simulink model "Vehicle_definitivo_validazione_2"  (R2025b)
settings: Solver=ode4  StartTime=0.0  StopTime=30  FixedStep=0.001  RelTol=1e-3
undefined symbols (not defined in the file): car, new_lotus_bump, new_lotus_roll, new_lotus_steer, posRef, rad, s, Tau_1, Tau_2, Tau_3, Tau_4, yawRef
libraries: aerolibconvert2 x28, simulink_extras x16, simulink x12, slpidlib x2, mpclib x1
(part 10 of 13)

== system Vehicle_definitivo_validazione_2/Torque Vectoring/Vehicle/Chassis/kinematics/FR ==
  note: mettere 2d su cmaber e toe
  Wheel_Travel : Inport
  Steer_Angle : Inport  Port=2
  Add : Sum
  Add1 : Sum  Inputs=+++
  Anti_dive : Lookup_n-D  NumberOfTableDimensions=1  BreakpointsForDimension1=[-20;-19;-18;-17;-16;-15;-14;-13;-12;-11;-10;-9;-8;-7;-6;-5;-4;-3;-2;-1;0;1;2;3;4;5;6;7;8;9;10;11;12;13;14;15;16;17;18;19;20;21;22;23;24;25;26;27;28;29;30;31;32;33;34;35;36;37;38;39;40;41;42;43;44;45;46;47;48;49;50;51;52;53;54;55;56;57;58;59;60;61;62;63;64;65;66;67;68;69;70;71;72;73;74;75]  Table=[53.85;54.03;54.22;54.4;54.59;54.77;54.96;55.15;55.34;55.53;55.72;55.92;56.11;56.31;56.5;56.7;56.9;57.1;57.3;57.5;57.71;57.91;58.12;58.32;58.53;58.74;58.95;59.16;59.38;59.59;59.81;60.03;60.24;60.46;60.69;60.91;61.13;61.36;61.59;61.81;62.04;62.28;62.51;62.74;62.98;63.22;63.46;63.7;63.94;64.18000000000001;64.43000000000001;64.68000000000001;64.92;65.17;65.43000000000001;65.68000000000001;65.94;66.19;66.45;66.72;66.98;67.23999999999999;67.51000000000001;67.78;68.05;68.31999999999999;68.59999999999999;68.87;69.15000000000001;69.43000000000001;69.72;70;70.29000000000001;70.58;70.87;71.16;71.45999999999999;71.75;72.05;72.36;72.66;72.97;73.28;73.59;73.91;74.22;74.54000000000001;74.86;75.19;75.52;75.84999999999999;76.18000000000001;76.51000000000001;76.84999999999999;77.19;77.54000000000001]/100  InternalRulePriority=Speed  RndMeth=Simplest
  Constant : Constant  Value=car.camber0_front
  Constant1 : Constant  Value=car.toe0_front
  Gain : Gain  Gain=0.222222
  IR : Lookup_n-D  NumberOfTableDimensions=1  BreakpointsForDimension1=[-20;-19;-18;-17;-16;-15;-14;-13;-12;-11;-10;-9;-8;-7;-6;-5;-4;-3;-2;-1;0;1;2;3;4;5;6;7;8;9;10;11;12;13;14;15;16;17;18;19;20;21;22;23;24;25;26;27;28;29;30;31;32;33;34;35;36;37;38;39;40;41;42;43;44;45;46;47;48;49;50;51;52;53;54;55;56;57;58;59;60;61;62;63;64;65;66;67;68;69;70;71;72;73;74;75]  Table=[0.556793;0.557414;0.558036;0.558659;0.559284;0.55991;0.5602240000000001;0.560538;0.561167;0.561167;0.561482;0.561798;0.562114;0.562114;0.562114;0.562114;0.562114;0.562114;0.562114;0.562114;0.561798;0.561798;0.561482;0.561482;0.561167;0.560852;0.560538;0.5602240000000001;0.55991;0.559284;0.558971;0.558347;0.558036;0.557414;0.557103;0.5564829999999999;0.555864;0.555247;0.554631;0.554017;0.553403;0.552792;0.552181;0.551572;0.550661;0.550055;0.549451;0.548546;0.547945;0.547046;0.546448;0.545554;0.544662;0.543774;0.543183;0.542299;0.541419;0.540541;0.539665;0.538793;0.537924;0.537057;0.536193;0.535332;0.534474;0.533618;0.532765;0.531915;0.531067;0.529942;0.529101;0.528262;0.527426;0.526593;0.525486;0.524659;0.523834;0.522739;0.521921;0.521105;0.5202909999999999;0.519211;0.5184029999999999;0.517598;0.516529;0.51573;0.514933;0.514139;0.513084;0.5122949999999999;0.511509;0.510725;0.509944;0.509165;0.508388;0.507614]  InternalRulePriority=Speed  RndMeth=Simplest
  camber : Lookup_n-D  NumberOfTableDimensions=1  BreakpointsForDimension1=[-20;-19;-18;-17;-16;-15;-14;-13;-12;-11;-10;-9;-8;-7;-6;-5;-4;-3;-2;-1;0;1;2;3;4;5;6;7;8;9;10;11;12;13;14;15;16;17;18;19;20;21;22;23;24;25;26;27;28;29;30;31;32;33;34;35;36;37;38;39;40;41;42;43;44;45;46;47;48;49;50;51;52;53;54;55;56;57;58;59;60;61;62;63;64;65;66;67;68;69;70;71;72;73;74;75]  Table=[0.17;0.13;0.08;0.04;-0.01;-0.05;-0.1;-0.15;-0.19;-0.24;-0.29;-0.33;-0.38;-0.42;-0.47;-0.52;-0.5600000000000001;-0.61;-0.66;-0.7;-0.75;-0.8;-0.84;-0.89;-0.9399999999999999;-0.98;-1.03;-1.08;-1.13;-1.17;-1.22;-1.27;-1.31;-1.36;-1.41;-1.46;-1.5;-1.55;-1.6;-1.65;-1.7;-1.74;-1.79;-1.84;-1.89;-1.94;-1.99;-2.03;-2.08;-2.13;-2.18;-2.23;-2.28;-2.33;-2.38;-2.42;-2.47;-2.52;-2.57;-2.62;-2.67;-2.72;-2.77;-2.82;-2.87;-2.92;-2.97;-3.02;-3.07;-3.12;-3.17;-3.23;-3.28;-3.33;-3.38;-3.43;-3.48;-3.53;-3.58;-3.64;-3.69;-3.74;-3.79;-3.84;-3.9;-3.95;-4;-4.05;-4.11;-4.16;-4.21;-4.27;-4.32;-4.37;-4.43;-4.48]+0.75  InternalRulePriority=Speed  RndMeth=Simplest
  steer vs toe : Lookup_n-D  NumberOfTableDimensions=1  BreakpointsForDimension1=new_lotus_steer.rack_travel  Table=new_lotus_steer.toe_angle_LHS  InternalRulePriority=Speed  RndMeth=Simplest
  toe : Lookup_n-D  NumberOfTableDimensions=1  BreakpointsForDimension1=[-20;-19;-18;-17;-16;-15;-14;-13;-12;-11;-10;-9;-8;-7;-6;-5;-4;-3;-2;-1;0;1;2;3;4;5;6;7;8;9;10;11;12;13;14;15;16;17;18;19;20;21;22;23;24;25;26;27;28;29;30;31;32;33;34;35;36;37;38;39;40;41;42;43;44;45;46;47;48;49;50;51;52;53;54;55;56;57;58;59;60;61;62;63;64;65;66;67;68;69;70;71;72;73;74;75]  Table=new_lotus_bump.front_LHS.toe  InternalRulePriority=Speed  RndMeth=Simplest
  wheelbase_change : Lookup_n-D  NumberOfTableDimensions=1  BreakpointsForDimension1=[-20;-19;-18;-17;-16;-15;-14;-13;-12;-11;-10;-9;-8;-7;-6;-5;-4;-3;-2;-1;0;1;2;3;4;5;6;7;8;9;10;11;12;13;14;15;16;17;18;19;20;21;22;23;24;25;26;27;28;29;30;31;32;33;34;35;36;37;38;39;40;41;42;43;44;45;46;47;48;49;50;51;52;53;54;55;56;57;58;59;60;61;62;63;64;65;66;67;68;69;70;71;72;73;74;75]  Table=[0.68000000000000005;0.65000000000000002;0.60999999999999999;0.56999999999999995;0.54000000000000004;0.5;0.46999999999999997;0.42999999999999999;0.40000000000000002;0.35999999999999999;0.33000000000000002;0.28999999999999998;0.26000000000000001;0.23000000000000001;0.19;0.16;0.13;0.089999999999999997;0.059999999999999998;0.029999999999999999;0;-0.029999999999999999;-0.059999999999999998;-0.089999999999999997;-0.12;-0.14999999999999999;-0.17999999999999999;-0.20999999999999999;-0.23999999999999999;-0.27000000000000002;-0.29999999999999999;-0.32000000000000001;-0.34999999999999998;-0.38;-0.40000000000000002;-0.42999999999999999;-0.46000000000000002;-0.47999999999999998;-0.51000000000000001;-0.53000000000000003;-0.56000000000000005;-0.57999999999999996;-0.60999999999999999;-0.63;-0.65000000000000002;-0.68000000000000005;-0.69999999999999996;-0.71999999999999997;-0.73999999999999999;-0.76000000000000001;-0.79000000000000004;-0.81000000000000005;-0.82999999999999996;-0.84999999999999998;-0.87;-0.89000000000000001;-0.91000000000000003;-0.92000000000000004;-0.93999999999999995;-0.95999999999999996;-0.97999999999999998;-0.98999999999999999;-1.01;-1.03;-1.04;-1.0600000000000001;-1.0700000000000001;-1.0900000000000001;-1.1000000000000001;-1.1200000000000001;-1.1299999999999999;-1.1399999999999999;-1.1499999999999999;-1.1699999999999999;-1.1799999999999999;-1.1899999999999999;-1.2;-1.21;-1.22;-1.23;-1.24;-1.25;-1.26;-1.26;-1.27;-1.28;-1.29;-1.29;-1.3;-1.3;-1.3100000000000001;-1.3100000000000001;-1.3100000000000001;-1.3200000000000001;-1.3200000000000001;-1.3200000000000001]/1000  InternalRulePriority=Speed  RndMeth=Simplest
  wb_FR : Outport
  AD_FR : Outport  Port=2
  IR_FR : Outport  Port=3
  Camber_FR : Outport  Port=4
  Toe_FR : Outport  Port=5
  wires:
  Wheel_Travel/1 -> Anti_dive/1, IR/1, toe/1, camber/1, wheelbase_change/1
  wheelbase_change/1 -> wb_FR/1
  Anti_dive/1 -> AD_FR/1
  IR/1 -> IR_FR/1
  camber/1 -> Add/2
  Constant/1 -> Add/1
  Add/1 -> Camber_FR/1
  Add1/1 -> Toe_FR/1
  Constant1/1 -> Add1/1
  toe/1 -> Add1/2
  steer vs toe/1 -> Add1/3  "toe_FR"
  Gain/1 -> steer vs toe/1
  Steer_Angle/1 -> Gain/1

== system Vehicle_definitivo_validazione_2/Torque Vectoring/Vehicle/Chassis/kinematics/RL ==
  Wheel_Travel : Inport
  Add : Sum
  Add2 : Sum
  Anti_squat : Lookup_n-D  NumberOfTableDimensions=1  BreakpointsForDimension1=[-20;-19;-18;-17;-16;-15;-14;-13;-12;-11;-10;-9;-8;-7;-6;-5;-4;-3;-2;-1;0;1;2;3;4;5;6;7;8;9;10;11;12;13;14;15;16;17;18;19;20;21;22;23;24;25;26;27;28;29;30;31;32;33;34;35;36;37;38;39;40;41;42;43;44;45;46;47;48;49;50;51;52;53;54;55;56;57;58;59;60;61;62;63;64;65;66;67;68;69;70;71;72;73;74;75]  Table=[53.82;53.82;53.82;53.82;53.82;53.82;53.82;53.82;53.82;53.82;53.83;53.83;53.83;53.83;53.84;53.84;53.84;53.85;53.85;53.86;53.86;53.87;53.87;53.88;53.88;53.89;53.9;53.9;53.91;53.92;53.92;53.93;53.94;53.95;53.95;53.96;53.97;53.98;53.99;54;54.01;54.01;54.02;54.03;54.04;54.05;54.06;54.07;54.08;54.09;54.1;54.11;54.12;54.13;54.15;54.16;54.17;54.18;54.19;54.2;54.21;54.22;54.23;54.24;54.25;54.27;54.28;54.29;54.3;54.31;54.32;54.33;54.34;54.35;54.36;54.37;54.38;54.39;54.4;54.41;54.42;54.43;54.44;54.45;54.46;54.47;54.48;54.49;54.49;54.5;54.51;54.52;54.52;54.53;54.54;54.54]/100  InternalRulePriority=Speed  RndMeth=Simplest
  Constant : Constant  Value=car.camber0_rear
  Constant2 : Constant  Value=car.toe0_rear
  Gain2 : Gain  Gain=-1
  IR : Lookup_n-D  NumberOfTableDimensions=1  BreakpointsForDimension1=[-20;-19;-18;-17;-16;-15;-14;-13;-12;-11;-10;-9;-8;-7;-6;-5;-4;-3;-2;-1;0;1;2;3;4;5;6;7;8;9;10;11;12;13;14;15;16;17;18;19;20;21;22;23;24;25;26;27;28;29;30;31;32;33;34;35;36;37;38;39;40;41;42;43;44;45;46;47;48;49;50;51;52;53;54;55;56;57;58;59;60;61;62;63;64;65;66;67;68;69;70;71;72;73;74;75]  Table=[0.7616000000000001;0.7616000000000001;0.7616000000000001;0.7616000000000001;0.7616000000000001;0.7616000000000001;0.7616000000000001;0.7622;0.7622;0.7628;0.7628;0.7634;0.7639;0.7645;0.7651;0.7657;0.7663;0.7669;0.7675;0.768;0.7692;0.7698;0.7704;0.7716;0.7722;0.7734;0.774;0.7746;0.7758;0.7764;0.7776;0.7782;0.7794;0.78;0.7813;0.7819;0.7831;0.7837;0.7849;0.7855;0.7868000000000001;0.7874;0.7886;0.7893;0.7905;0.7911;0.7917999999999999;0.793;0.7937;0.7943;0.7949000000000001;0.7962;0.7968;0.7974;0.7981;0.7987;0.7994;0.8;0.8;0.8006;0.8013;0.8013;0.8018999999999999;0.8018999999999999;0.8026;0.8026;0.8026;0.8026;0.8026;0.8026;0.8026;0.8018999999999999;0.8018999999999999;0.8013;0.8006;0.8;0.7994;0.7987;0.7974;0.7968;0.7955;0.7943;0.7924;0.7911;0.7893;0.7874;0.7849;0.7831;0.7806;0.7776;0.7752;0.7722;0.7685999999999999;0.7651;0.7616000000000001;0.7576000000000001]  InternalRulePriority=Speed  RndMeth=Simplest
  camber : Lookup_n-D  NumberOfTableDimensions=1  BreakpointsForDimension1=[-20;-19;-18;-17;-16;-15;-14;-13;-12;-11;-10;-9;-8;-7;-6;-5;-4;-3;-2;-1;0;1;2;3;4;5;6;7;8;9;10;11;12;13;14;15;16;17;18;19;20;21;22;23;24;25;26;27;28;29;30;31;32;33;34;35;36;37;38;39;40;41;42;43;44;45;46;47;48;49;50;51;52;53;54;55;56;57;58;59;60;61;62;63;64;65;66;67;68;69;70;71;72;73;74;75]  Table=[0.79000000000000004;0.75;0.70999999999999996;0.67000000000000004;0.63;0.58999999999999997;0.55000000000000004;0.51000000000000001;0.46999999999999997;0.42999999999999999;0.39000000000000001;0.34999999999999998;0.31;0.27000000000000002;0.23999999999999999;0.20000000000000001;0.16;0.12;0.080000000000000002;0.040000000000000001;0;-0.040000000000000001;-0.080000000000000002;-0.12;-0.16;-0.20000000000000001;-0.23999999999999999;-0.27000000000000002;-0.31;-0.34999999999999998;-0.39000000000000001;-0.42999999999999999;-0.46999999999999997;-0.51000000000000001;-0.55000000000000004;-0.58999999999999997;-0.63;-0.67000000000000004;-0.70999999999999996;-0.75;-0.79000000000000004;-0.82999999999999996;-0.85999999999999999;-0.90000000000000002;-0.93999999999999995;-0.97999999999999998;-1.02;-1.0600000000000001;-1.1000000000000001;-1.1399999999999999;-1.1799999999999999;-1.22;-1.26;-1.3;-1.3400000000000001;-1.3799999999999999;-1.4199999999999999;-1.46;-1.5;-1.54;-1.5800000000000001;-1.6200000000000001;-1.6599999999999999;-1.7;-1.74;-1.78;-1.8200000000000001;-1.8600000000000001;-1.8999999999999999;-1.9399999999999999;-1.98;-2.02;-2.0699999999999998;-2.1099999999999999;-2.1499999999999999;-2.1899999999999999;-2.23;-2.27;-2.3100000000000001;-2.3500000000000001;-2.3900000000000001;-2.4399999999999999;-2.48;-2.52;-2.5600000000000001;-2.6000000000000001;-2.6400000000000001;-2.6899999999999999;-2.73;-2.77;-2.8100000000000001;-2.8500000000000001;-2.8999999999999999;-2.9399999999999999;-2.98;-3.02]  InternalRulePriority=Speed  RndMeth=Simplest
  toe : Lookup_n-D  NumberOfTableDimensions=1  BreakpointsForDimension1=new_lotus_bump.wheeltravel  Table=new_lotus_bump.rear_LHS.toe  InternalRulePriority=Speed  RndMeth=Simplest
  wheelbase_change : Lookup_n-D  NumberOfTableDimensions=1  BreakpointsForDimension1=[-20;-19;-18;-17;-16;-15;-14;-13;-12;-11;-10;-9;-8;-7;-6;-5;-4;-3;-2;-1;0;1;2;3;4;5;6;7;8;9;10;11;12;13;14;15;16;17;18;19;20;21;22;23;24;25;26;27;28;29;30;31;32;33;34;35;36;37;38;39;40;41;42;43;44;45;46;47;48;49;50;51;52;53;54;55;56;57;58;59;60;61;62;63;64;65;66;67;68;69;70;71;72;73;74;75]  Table=[-2.1899999999999999;-2.0800000000000001;-1.97;-1.8600000000000001;-1.74;-1.6299999999999999;-1.52;-1.4099999999999999;-1.3;-1.1899999999999999;-1.0800000000000001;-0.96999999999999997;-0.85999999999999999;-0.75;-0.65000000000000002;-0.54000000000000004;-0.42999999999999999;-0.32000000000000001;-0.20999999999999999;-0.11;0;0.11;0.20999999999999999;0.32000000000000001;0.41999999999999998;0.53000000000000003;0.63;0.73999999999999999;0.83999999999999997;0.94999999999999996;1.05;1.1599999999999999;1.26;1.3600000000000001;1.47;1.5700000000000001;1.6699999999999999;1.77;1.8700000000000001;1.98;2.0800000000000001;2.1800000000000002;2.2799999999999998;2.3799999999999999;2.48;2.5800000000000001;2.6800000000000002;2.7799999999999998;2.8799999999999999;2.9700000000000002;3.0699999999999998;3.1699999999999999;3.27;3.3700000000000001;3.46;3.5600000000000001;3.6600000000000001;3.7599999999999998;3.8500000000000001;3.9500000000000002;4.04;4.1399999999999997;4.2400000000000002;4.3300000000000001;4.4299999999999997;4.5199999999999996;4.6100000000000003;4.71;4.7999999999999998;4.9000000000000004;4.9900000000000002;5.0800000000000001;5.1799999999999997;5.2699999999999996;5.3600000000000003;5.4500000000000002;5.5499999999999998;5.6399999999999997;5.7300000000000004;5.8200000000000003;5.9100000000000001;6;6.0899999999999999;6.1799999999999997;6.2699999999999996;6.3600000000000003;6.4500000000000002;6.54;6.6299999999999999;6.7199999999999998;6.8099999999999996;6.9000000000000004;6.9900000000000002;7.0700000000000003;7.1600000000000001;7.25]/1000  InternalRulePriority=Speed  RndMeth=Simplest
  wb_RL : Outport
  AS_RL : Outport  Port=2
  IR_RL : Outport  Port=3
  Camber_RL : Outport  Port=4
  Toe_RL : Outport  Port=5
  wires:
  Wheel_Travel/1 -> Anti_squat/1, wheelbase_change/1, IR/1, toe/1, camber/1
  wheelbase_change/1 -> wb_RL/1
  Anti_squat/1 -> AS_RL/1
  IR/1 -> IR_RL/1
  Add/1 -> Camber_RL/1
  Constant/1 -> Add/1
  camber/1 -> Add/2
  Constant2/1 -> Add2/1
  Add2/1 -> Toe_RL/1
  toe/1 -> Gain2/1
  Gain2/1 -> Add2/2

== system Vehicle_definitivo_validazione_2/Torque Vectoring/Vehicle/Chassis/kinematics/RR ==
  Wheel_Travel : Inport
  Add : Sum
  Add2 : Sum
  Anti_squat : Lookup_n-D  NumberOfTableDimensions=1  BreakpointsForDimension1=[-20;-19;-18;-17;-16;-15;-14;-13;-12;-11;-10;-9;-8;-7;-6;-5;-4;-3;-2;-1;0;1;2;3;4;5;6;7;8;9;10;11;12;13;14;15;16;17;18;19;20;21;22;23;24;25;26;27;28;29;30;31;32;33;34;35;36;37;38;39;40;41;42;43;44;45;46;47;48;49;50;51;52;53;54;55;56;57;58;59;60;61;62;63;64;65;66;67;68;69;70;71;72;73;74;75]  Table=[53.82;53.82;53.82;53.82;53.82;53.82;53.82;53.82;53.82;53.82;53.83;53.83;53.83;53.83;53.84;53.84;53.84;53.85;53.85;53.86;53.86;53.87;53.87;53.88;53.88;53.89;53.9;53.9;53.91;53.92;53.92;53.93;53.94;53.95;53.95;53.96;53.97;53.98;53.99;54;54.01;54.01;54.02;54.03;54.04;54.05;54.06;54.07;54.08;54.09;54.1;54.11;54.12;54.13;54.15;54.16;54.17;54.18;54.19;54.2;54.21;54.22;54.23;54.24;54.25;54.27;54.28;54.29;54.3;54.31;54.32;54.33;54.34;54.35;54.36;54.37;54.38;54.39;54.4;54.41;54.42;54.43;54.44;54.45;54.46;54.47;54.48;54.49;54.49;54.5;54.51;54.52;54.52;54.53;54.54;54.54]/100  InternalRulePriority=Speed  RndMeth=Simplest
  Constant : Constant  Value=car.camber0_rear
  Constant2 : Constant  Value=car.toe0_rear
  IR : Lookup_n-D  NumberOfTableDimensions=1  BreakpointsForDimension1=[-20;-19;-18;-17;-16;-15;-14;-13;-12;-11;-10;-9;-8;-7;-6;-5;-4;-3;-2;-1;0;1;2;3;4;5;6;7;8;9;10;11;12;13;14;15;16;17;18;19;20;21;22;23;24;25;26;27;28;29;30;31;32;33;34;35;36;37;38;39;40;41;42;43;44;45;46;47;48;49;50;51;52;53;54;55;56;57;58;59;60;61;62;63;64;65;66;67;68;69;70;71;72;73;74;75]  Table=[0.7616000000000001;0.7616000000000001;0.7616000000000001;0.7616000000000001;0.7616000000000001;0.7616000000000001;0.7616000000000001;0.7622;0.7622;0.7628;0.7628;0.7634;0.7639;0.7645;0.7651;0.7657;0.7663;0.7669;0.7675;0.768;0.7692;0.7698;0.7704;0.7716;0.7722;0.7734;0.774;0.7746;0.7758;0.7764;0.7776;0.7782;0.7794;0.78;0.7813;0.7819;0.7831;0.7837;0.7849;0.7855;0.7868000000000001;0.7874;0.7886;0.7893;0.7905;0.7911;0.7917999999999999;0.793;0.7937;0.7943;0.7949000000000001;0.7962;0.7968;0.7974;0.7981;0.7987;0.7994;0.8;0.8;0.8006;0.8013;0.8013;0.8018999999999999;0.8018999999999999;0.8026;0.8026;0.8026;0.8026;0.8026;0.8026;0.8026;0.8018999999999999;0.8018999999999999;0.8013;0.8006;0.8;0.7994;0.7987;0.7974;0.7968;0.7955;0.7943;0.7924;0.7911;0.7893;0.7874;0.7849;0.7831;0.7806;0.7776;0.7752;0.7722;0.7685999999999999;0.7651;0.7616000000000001;0.7576000000000001]  InternalRulePriority=Speed  RndMeth=Simplest
  camber : Lookup_n-D  NumberOfTableDimensions=1  BreakpointsForDimension1=[-20;-19;-18;-17;-16;-15;-14;-13;-12;-11;-10;-9;-8;-7;-6;-5;-4;-3;-2;-1;0;1;2;3;4;5;6;7;8;9;10;11;12;13;14;15;16;17;18;19;20;21;22;23;24;25;26;27;28;29;30;31;32;33;34;35;36;37;38;39;40;41;42;43;44;45;46;47;48;49;50;51;52;53;54;55;56;57;58;59;60;61;62;63;64;65;66;67;68;69;70;71;72;73;74;75]  Table=[0.79000000000000004;0.75;0.70999999999999996;0.67000000000000004;0.63;0.58999999999999997;0.55000000000000004;0.51000000000000001;0.46999999999999997;0.42999999999999999;0.39000000000000001;0.34999999999999998;0.31;0.27000000000000002;0.23999999999999999;0.20000000000000001;0.16;0.12;0.080000000000000002;0.040000000000000001;0;-0.040000000000000001;-0.080000000000000002;-0.12;-0.16;-0.20000000000000001;-0.23999999999999999;-0.27000000000000002;-0.31;-0.34999999999999998;-0.39000000000000001;-0.42999999999999999;-0.46999999999999997;-0.51000000000000001;-0.55000000000000004;-0.58999999999999997;-0.63;-0.67000000000000004;-0.70999999999999996;-0.75;-0.79000000000000004;-0.82999999999999996;-0.85999999999999999;-0.90000000000000002;-0.93999999999999995;-0.97999999999999998;-1.02;-1.0600000000000001;-1.1000000000000001;-1.1399999999999999;-1.1799999999999999;-1.22;-1.26;-1.3;-1.3400000000000001;-1.3799999999999999;-1.4199999999999999;-1.46;-1.5;-1.54;-1.5800000000000001;-1.6200000000000001;-1.6599999999999999;-1.7;-1.74;-1.78;-1.8200000000000001;-1.8600000000000001;-1.8999999999999999;-1.9399999999999999;-1.98;-2.02;-2.0699999999999998;-2.1099999999999999;-2.1499999999999999;-2.1899999999999999;-2.23;-2.27;-2.3100000000000001;-2.3500000000000001;-2.3900000000000001;-2.4399999999999999;-2.48;-2.52;-2.5600000000000001;-2.6000000000000001;-2.6400000000000001;-2.6899999999999999;-2.73;-2.77;-2.8100000000000001;-2.8500000000000001;-2.8999999999999999;-2.9399999999999999;-2.98;-3.02]  InternalRulePriority=Speed  RndMeth=Simplest
  toe : Lookup_n-D  NumberOfTableDimensions=1  BreakpointsForDimension1=new_lotus_bump.wheeltravel  Table=new_lotus_bump.rear_LHS.toe  InternalRulePriority=Speed  RndMeth=Simplest
  wheelbase_change : Lookup_n-D  NumberOfTableDimensions=1  BreakpointsForDimension1=[-20;-19;-18;-17;-16;-15;-14;-13;-12;-11;-10;-9;-8;-7;-6;-5;-4;-3;-2;-1;0;1;2;3;4;5;6;7;8;9;10;11;12;13;14;15;16;17;18;19;20;21;22;23;24;25;26;27;28;29;30;31;32;33;34;35;36;37;38;39;40;41;42;43;44;45;46;47;48;49;50;51;52;53;54;55;56;57;58;59;60;61;62;63;64;65;66;67;68;69;70;71;72;73;74;75]  Table=[-2.1899999999999999;-2.0800000000000001;-1.97;-1.8600000000000001;-1.74;-1.6299999999999999;-1.52;-1.4099999999999999;-1.3;-1.1899999999999999;-1.0800000000000001;-0.96999999999999997;-0.85999999999999999;-0.75;-0.65000000000000002;-0.54000000000000004;-0.42999999999999999;-0.32000000000000001;-0.20999999999999999;-0.11;0;0.11;0.20999999999999999;0.32000000000000001;0.41999999999999998;0.53000000000000003;0.63;0.73999999999999999;0.83999999999999997;0.94999999999999996;1.05;1.1599999999999999;1.26;1.3600000000000001;1.47;1.5700000000000001;1.6699999999999999;1.77;1.8700000000000001;1.98;2.0800000000000001;2.1800000000000002;2.2799999999999998;2.3799999999999999;2.48;2.5800000000000001;2.6800000000000002;2.7799999999999998;2.8799999999999999;2.9700000000000002;3.0699999999999998;3.1699999999999999;3.27;3.3700000000000001;3.46;3.5600000000000001;3.6600000000000001;3.7599999999999998;3.8500000000000001;3.9500000000000002;4.04;4.1399999999999997;4.2400000000000002;4.3300000000000001;4.4299999999999997;4.5199999999999996;4.6100000000000003;4.71;4.7999999999999998;4.9000000000000004;4.9900000000000002;5.0800000000000001;5.1799999999999997;5.2699999999999996;5.3600000000000003;5.4500000000000002;5.5499999999999998;5.6399999999999997;5.7300000000000004;5.8200000000000003;5.9100000000000001;6;6.0899999999999999;6.1799999999999997;6.2699999999999996;6.3600000000000003;6.4500000000000002;6.54;6.6299999999999999;6.7199999999999998;6.8099999999999996;6.9000000000000004;6.9900000000000002;7.0700000000000003;7.1600000000000001;7.25]/1000  InternalRulePriority=Speed  RndMeth=Simplest
  wb_RR : Outport
  AS_RR : Outport  Port=2
  IR_RR : Outport  Port=3
  Camber_RR : Outport  Port=4
  Toe_RR : Outport  Port=5
  wires:
  Wheel_Travel/1 -> Anti_squat/1, wheelbase_change/1, IR/1, camber/1, toe/1
  wheelbase_change/1 -> wb_RR/1
  Anti_squat/1 -> AS_RR/1
  IR/1 -> IR_RR/1
  Add/1 -> Camber_RR/1
  Constant/1 -> Add/1
  camber/1 -> Add/2
  Constant2/1 -> Add2/1
  Add2/1 -> Toe_RR/1
  toe/1 -> Add2/2

== system Vehicle_definitivo_validazione_2/Torque Vectoring/Vehicle/Chassis/kinematics/Subsystem ==
  Heave_F : Inport
  Roll_F : Inport  Port=2
  Add : Sum
  Constant : Constant  Value=car.tf
  Constant1 : Constant  Value=car.tf
  Divide : Product  Inputs=*/
  Gain : Gain  Gain=-1
  H_rc : Lookup_n-D  BreakpointsForDimension1=[1:3]  BreakpointsForDimension2=[1:3]  InternalRulePriority=Speed  RndMeth=Simplest
      settings: InputPortMap=u0,u1
  Radians to Degrees : simulink_extras/Transformations/Radians to Degrees
  Tan : Trigonometry  Operator=atan
  track_change : Lookup_n-D  NumberOfTableDimensions=1  BreakpointsForDimension1=new_lotus_roll.roll_angle  Table=new_lotus_roll.front_LHS.half_track_change/1000  InternalRulePriority=Speed  RndMeth=Simplest
  h_rc_f : Outport
  tf : Outport  Port=2
  wires:
  Heave_F/1 -> H_rc/1
  track_change/1 -> Add/1  "track_change"
  Constant/1 -> Add/2
  Add/1 -> tf/1  "tf"
  H_rc/1 -> h_rc_f/1  "h_rc_f"
  Roll_F/1 -> Divide/1
  Divide/1 -> Tan/1
  Tan/1 -> Radians to Degrees/1
  Gain/1 -> track_change/1, H_rc/2
  Constant1/1 -> Divide/2
  Radians to Degrees/1 -> Gain/1

== system Vehicle_definitivo_validazione_2/Torque Vectoring/Vehicle/Chassis/kinematics/Subsystem1 ==
  Heave_R : Inport
  Roll_R : Inport  Port=2
  Add : Sum
  Constant : Constant  Value=car.tr
  Constant1 : Constant  Value=car.tr
  Divide : Product  Inputs=*/
  Gain : Gain  Gain=-1
  H_rc : Lookup_n-D  BreakpointsForDimension1=[1:3]  BreakpointsForDimension2=[1:3]  InternalRulePriority=Speed  RndMeth=Simplest
      settings: InputPortMap=u0,u1
  Radians to Degrees : simulink_extras/Transformations/Radians to Degrees
  Tan : Trigonometry  Operator=atan
  track_change : Lookup_n-D  NumberOfTableDimensions=1  BreakpointsForDimension1=new_lotus_roll.roll_angle  Table=new_lotus_roll.rear_LHS.half_track_change/1000  InternalRulePriority=Speed  RndMeth=Simplest
  h_rc_r : Outport
  tr : Outport  Port=2
  wires:
  track_change/1 -> Add/1  "track_change"
  Constant/1 -> Add/2
  H_rc/1 -> h_rc_r/1  "h_rc_r"
  Roll_R/1 -> Divide/1
  Heave_R/1 -> H_rc/1
  Divide/1 -> Tan/1
  Add/1 -> tr/1  "tr"
  Gain/1 -> track_change/1, H_rc/2
  Constant1/1 -> Divide/2
  Tan/1 -> Radians to Degrees/1
  Radians to Degrees/1 -> Gain/1

== system Vehicle_definitivo_validazione_2/Torque Vectoring/Vehicle/Powertrain/pwt con clutch/Engine ==
  w_ICE : Inport
  tps : Inport  Port=2
  1-D Lookup Table : Lookup_n-D  NumberOfTableDimensions=1  BreakpointsForDimension1=[0 car.limitatore car.limitatore+300]  Table=[1 1 0]  InternalRulePriority=Speed  RndMeth=Simplest
  2-D Lookup Table : Lookup_n-D  BreakpointsForDimension1=[0;4000;4500;5000;5500;6000;6500;7000;7500;8000;8500;9000;9500;10000;10500;11000;11500;12000]  BreakpointsForDimension2=[0;0.20000000000000001;0.25;0.29999999999999999;0.34999999999999998;0.40000000000000002;0.45000000000000001;0.5;0.59999999999999998;0.69999999999999996;0.80000000000000004;1]  Table=car.engine.lut  InternalRulePriority=Speed  RndMeth=Simplest
      settings: InputPortMap=u0,u1
  Limiter : Saturate  UpperLimit=12500  LowerLimit=4000
  Product : Product
  T_ICE : Outport
  wires:
  tps/1 -> 2-D Lookup Table/2
  Limiter/1 -> 2-D Lookup Table/1
  w_ICE/1 -> Limiter/1, 1-D Lookup Table/1
  1-D Lookup Table/1 -> Product/1
  2-D Lookup Table/1 -> Product/2
  Product/1 -> T_ICE/1

== system Vehicle_definitivo_validazione_2/Torque Vectoring/Vehicle/Powertrain/pwt con clutch/Transmission ==
  T_ICE : Inport
  gear : Inport  Port=2
  1-D Lookup Table2 : Lookup_n-D  NumberOfTableDimensions=1  BreakpointsForDimension1=[1;2;3;4]  Table=[Tau_1; Tau_2; Tau_3; Tau_4]  InternalRulePriority=Speed  RndMeth=Simplest
  Gain1 : Gain  Gain=car.eta_pwt
  Product1 : Product
  T_rear : Outport
  wires:
  Gain1/1 -> T_rear/1
  Product1/1 -> Gain1/1
  T_ICE/1 -> Product1/2
  1-D Lookup Table2/1 -> Product1/1
  gear/1 -> 1-D Lookup Table2/1

== system Vehicle_definitivo_validazione_2/Torque Vectoring/Vehicle/Powertrain/pwt senza clutch/Engine ==
  w_ICE : Inport
  tps : Inport  Port=2
  1-D Lookup Table : Lookup_n-D  NumberOfTableDimensions=1  BreakpointsForDimension1=[0 car.limitatore car.limitatore+300]  Table=[1 1 0]  InternalRulePriority=Speed  RndMeth=Simplest
  2-D Lookup Table : Lookup_n-D  BreakpointsForDimension1=[0;4000;4500;5000;5500;6000;6500;7000;7500;8000;8500;9000;9500;10000;10500;11000;11500;12000]  BreakpointsForDimension2=[0;0.20000000000000001;0.25;0.29999999999999999;0.34999999999999998;0.40000000000000002;0.45000000000000001;0.5;0.59999999999999998;0.69999999999999996;0.80000000000000004;1]  Table=car.engine.lut  InternalRulePriority=Speed  RndMeth=Simplest
      settings: InputPortMap=u0,u1
  Limiter : Saturate  UpperLimit=12500  LowerLimit=4000
  Product : Product
  T_ICE : Outport
  wires:
  tps/1 -> 2-D Lookup Table/2
  Limiter/1 -> 2-D Lookup Table/1
  w_ICE/1 -> Limiter/1, 1-D Lookup Table/1
  1-D Lookup Table/1 -> Product/1
  2-D Lookup Table/1 -> Product/2
  Product/1 -> T_ICE/1

== system Vehicle_definitivo_validazione_2/Torque Vectoring/Vehicle/Powertrain/pwt senza clutch/Transmission ==
  T_ICE : Inport
  gear : Inport  Port=2
  1-D Lookup Table2 : Lookup_n-D  NumberOfTableDimensions=1  BreakpointsForDimension1=[1;2;3;4]  Table=[Tau_1; Tau_2; Tau_3; Tau_4]  InternalRulePriority=Speed  RndMeth=Simplest
  Gain1 : Gain  Gain=car.eta_pwt
  Product1 : Product
  T_rear : Outport
  wires:
  Gain1/1 -> T_rear/1
  Product1/1 -> Gain1/1
  T_ICE/1 -> Product1/2
  1-D Lookup Table2/1 -> Product1/1
  gear/1 -> 1-D Lookup Table2/1

== system Vehicle_definitivo_validazione_2/Torque Vectoring/Vehicle/Powertrain con differenziale1/pwt con clutch/Engine ==
  w_ICE : Inport
  tps : Inport  Port=2
  1-D Lookup Table : Lookup_n-D  NumberOfTableDimensions=1  BreakpointsForDimension1=[0 car.limitatore car.limitatore+300]  Table=[1 1 0]  InternalRulePriority=Speed  RndMeth=Simplest
  2-D Lookup Table : Lookup_n-D  BreakpointsForDimension1=[0;4000;4500;5000;5500;6000;6500;7000;7500;8000;8500;9000;9500;10000;10500;11000;11500;12000]  BreakpointsForDimension2=[0;0.20000000000000001;0.25;0.29999999999999999;0.34999999999999998;0.40000000000000002;0.45000000000000001;0.5;0.59999999999999998;0.69999999999999996;0.80000000000000004;1]  Table=car.engine.lut  InternalRulePriority=Speed  RndMeth=Simplest
      settings: InputPortMap=u0,u1
  Limiter : Saturate  UpperLimit=12500  LowerLimit=4000
  Product : Product
  T_ICE : Outport
  wires:
  Product/1 -> T_ICE/1
  2-D Lookup Table/1 -> Product/2
  1-D Lookup Table/1 -> Product/1
  w_ICE/1 -> 1-D Lookup Table/1, Limiter/1
  Limiter/1 -> 2-D Lookup Table/1
  tps/1 -> 2-D Lookup Table/2

== system Vehicle_definitivo_validazione_2/Torque Vectoring/Vehicle/Powertrain con differenziale1/pwt con clutch/Transmission ==
  T_ICE : Inport
  gear : Inport  Port=2
  1-D Lookup Table2 : Lookup_n-D  NumberOfTableDimensions=1  BreakpointsForDimension1=[1;2;3;4]  Table=[Tau_1; Tau_2; Tau_3; Tau_4]  InternalRulePriority=Speed  RndMeth=Simplest
  Gain1 : Gain  Gain=car.eta_pwt
  Product1 : Product
  T_rear : Outport
  wires:
  gear/1 -> 1-D Lookup Table2/1
  1-D Lookup Table2/1 -> Product1/1
  T_ICE/1 -> Product1/2
  Product1/1 -> Gain1/1
  Gain1/1 -> T_rear/1

== system Vehicle_definitivo_validazione_2/Torque Vectoring/Vehicle/Powertrain con differenziale1/pwt senza clutch/Engine ==
  w_ICE : Inport
  tps : Inport  Port=2
  1-D Lookup Table : Lookup_n-D  NumberOfTableDimensions=1  BreakpointsForDimension1=[0 car.limitatore car.limitatore+300]  Table=[1 1 0]  InternalRulePriority=Speed  RndMeth=Simplest
  2-D Lookup Table : Lookup_n-D  BreakpointsForDimension1=[0;4000;4500;5000;5500;6000;6500;7000;7500;8000;8500;9000;9500;10000;10500;11000;11500;12000]  BreakpointsForDimension2=[0;0.20000000000000001;0.25;0.29999999999999999;0.34999999999999998;0.40000000000000002;0.45000000000000001;0.5;0.59999999999999998;0.69999999999999996;0.80000000000000004;1]  Table=car.engine.lut  InternalRulePriority=Speed  RndMeth=Simplest
      settings: InputPortMap=u0,u1
  Limiter : Saturate  UpperLimit=12500  LowerLimit=4000
  Product : Product
  T_ICE : Outport
  wires:
  Product/1 -> T_ICE/1
  2-D Lookup Table/1 -> Product/2
  1-D Lookup Table/1 -> Product/1
  w_ICE/1 -> 1-D Lookup Table/1, Limiter/1
  Limiter/1 -> 2-D Lookup Table/1
  tps/1 -> 2-D Lookup Table/2

== system Vehicle_definitivo_validazione_2/Torque Vectoring/Vehicle/Powertrain con differenziale1/pwt senza clutch/Transmission ==
  T_ICE : Inport
  gear : Inport  Port=2
  1-D Lookup Table2 : Lookup_n-D  NumberOfTableDimensions=1  BreakpointsForDimension1=[1;2;3;4]  Table=[Tau_1; Tau_2; Tau_3; Tau_4]  InternalRulePriority=Speed  RndMeth=Simplest
  Gain1 : Gain  Gain=car.eta_pwt
  Product1 : Product
  T_rear : Outport
  wires:
  gear/1 -> 1-D Lookup Table2/1
  1-D Lookup Table2/1 -> Product1/1
  T_ICE/1 -> Product1/2
  Product1/1 -> Gain1/1
  Gain1/1 -> T_rear/1

== matlab function Vehicle_definitivo_validazione_2/Torque Vectoring/Vehicle Control Unit/Low Level Controller/MATLAB Function ==
  data: Fy input; Fz input; T_front input; T_target_FR output; car input; T_target_FL output
function [T_target_FR, T_target_FL] = fcn_DynamicSaturation(Fy, Fz, T_front, car)
    
    R = car.R; 
    tau = car.Tau_EM; 
    eta = 1.0; % EFFICIENZA IDEALE
    mu_est = 1.8; 
    T_target_FR = 0.0;
    T_target_FL = 0.0;

    % =========================================================
    % A) CALCOLO LIMITE RUOTA DESTRA (FR - Indice 1)
    % =========================================================
    F_tot_max_FR = mu_est * Fz(1);
    Fx_max_FR = sqrt(max((F_tot_max_FR^2 - Fy(1)^2), 0));
    T_grip_motore_FR = (Fx_max_FR * R) / (tau * eta);
    
    % =========================================================
    % B) CALCOLO LIMITE RUOTA SINISTRA (FL - Indice 2)
    % =========================================================
    F_tot_max_FL = mu_est * Fz(2);
    Fx_max_FL = sqrt(max((F_tot_max_FL^2 - Fy(2)^2), 0));
    T_grip_motore_FL = (Fx_max_FL * R) / (tau * eta);
    
    % =========================================================
    % C) SATURAZIONE DINAMICA E ASSEGNAZIONE
    % =========================================================
    T_target_FR = max(min(T_front(1), T_grip_motore_FR), -T_grip_motore_FR);
    T_target_FL = max(min(T_front(2), T_grip_motore_FL), -T_grip_motore_FL);
    
end

== matlab function Vehicle_definitivo_validazione_2/Torque Vectoring/Vehicle/Powertrain/Electric Motor/MATLAB Function1 ==
  data: T_target input; T_actual_FR output; T_max_pos_FR input; T_max_neg_FR input; T_max_pos_FL input; T_max_neg_FL input; T_actual_FL output
function [T_actual_FR, T_actual_FL] = fcn_Saturation(T_target, T_max_pos_FR, T_max_neg_FR, T_max_pos_FL, T_max_neg_FL)
    
    T_actual_FR=0;
    T_actual_FL=0;
    
    T_actual_FR = max(min(T_target(1), T_max_pos_FR), T_max_neg_FR);
    T_actual_FL = max(min(T_target(2), T_max_pos_FL), T_max_neg_FL);

end

== matlab function Vehicle_definitivo_validazione_2/Senza relaxation/Vehicle/Powertrain/pwt con clutch/MATLAB Function4 ==
  data: u input; next_gear output; tps input; bps input; current_gear input; shift_timer_in input; shift_timer_out output; torque_mult output
function [next_gear, shift_timer_out, torque_mult] = Gearbox_ECU(u, tps, bps, current_gear, shift_timer_in)
   
    dt = 0.001;               
    shift_duration = 0.030;   
    nGearMax = 4;             
    
    v_thresh_up   = [0, 24.9444, 29.1, inf]; 
    v_thresh_down = [0, 18, 26.5, 29.5];
    
    % Inizializzazione sicura
    % if current_gear == 0
    %     current_gear = 2; % Partenza in 2° marcia
    % end
    
    next_gear = current_gear;
    
    if shift_timer_in > 0
        torque_mult = 0;                           
        shift_timer_out = shift_timer_in - dt;     
    else
        torque_mult = 1;                           
        shift_timer_out = 0;                       
        if current_gear < nGearMax && u >= v_thresh_up(current_gear) && tps > 0 && bps == 0
            next_gear = current_gear + 1;
            shift_timer_out = shift_duration;                  
        elseif current_gear > 1 && u <= v_thresh_down(current_gear) && (bps > 0 || tps == 0)
            next_gear = current_gear - 1;
            shift_timer_out = shift_duration;      
        end
    end
end

== matlab function Vehicle_definitivo_validazione_2/Senza relaxation/Vehicle/Powertrain/pwt senza clutch/Differential ==
  data: T_rear input; T_RR output; w_RR input; w_RL input; T_RL output; car input
function [T_RR, T_RL] = fcn_Salisbury_LSD(T_rear, w_RR, w_RL, car)
   
    % Coefficienti di smoothing (Stabilità Simulink)
    k_blend = 10; 
    k_slip  = 5; 
    
    % --- 2. TRANSIZIONE POWER-ON / POWER-OFF (Senza IF) ---
    w_blend = 0.5 * (1 + tanh(k_blend * T_rear));
    mu_active = car.mu_Poff + (car.mu_Pon - car.mu_Poff) * w_blend;
    
    % --- 3. CALCOLO CAPACITÀ DI BLOCCAGGIO (Mf_max) ---
    T_ramps = mu_active * abs(T_rear);
    Mf_max = max(car.Mf_preload, T_ramps); 
    
    % --- 4. APPLICAZIONE COPPIA ATTRITO (Modello Continuo) ---
    delta_w = w_RR - w_RL; 
    T_lock = Mf_max * tanh(k_slip * delta_w);
    
    % --- 5. RIPARTIZIONE FINALE ---
    % Se w_RR è maggiore (delta_w > 0, T_lock > 0), tolgo a RR e do a RL
    T_RR = (T_rear / 2) - T_lock;
    T_RL = (T_rear / 2) + T_lock;
end

== matlab function Vehicle_definitivo_validazione_2/Driver in the Loop/Vehicle/Chassis/MATLAB Function4 ==
  data: gear input; car input; Jr_tot output
function Jr_tot  = Jr(gear, car)

if gear == 1 
    Jr_tot = car.Jr_tot_1;
elseif gear == 2 
    Jr_tot = car.Jr_tot_2;
elseif gear == 3 
    Jr_tot = car.Jr_tot_3;
elseif gear == 4
    Jr_tot = car.Jr_tot_4;
else  
    Jr_tot = car.Jr_tot_0;
end

== matlab function Vehicle_definitivo_validazione_2/Driver in the Loop/Vehicle/Chassis/MATLAB Function5 ==
  data: x input; kin input; ax_prev input; ay_prev input; u input; dx output size=[14 1]; Jr_tot input; F_damp_in input; aero_coeffs input; car input; Fz output size=[4 1]; Drag output size=1; wheel_travel output size=[4 1]; susp_vel_ground output size=[4 1]; IR output size=[4 1]; corner_rh output size=[4 1]; tyre_deflection output; damping output
function [dx, Fz, Drag, wheel_travel, susp_vel_ground, IR, corner_rh, tyre_deflection, damping] = fcn_Ride_Model(x, kin, ax_prev, ay_prev, u, Jr_tot, F_damp_in, aero_coeffs, car)

    % --- 1. Estrazione degli Stati ---
    q  = x(1:7);      % [z_heave; theta_pitch; phi_roll; z_uFL; z_uFR; z_uRL; z_uRR]
    dq = x(8:14);     % Velocità
    damping = x(4);

    % --- 2. UNPACKING PARAMETRI DINAMICI ---  
    IR_FR = car.IR_spring_front;   IR_FL = car.IR_spring_front;
    IR_RR = car.IR_spring_rear;    IR_RL = car.IR_spring_rear;
    tf = car.tf;      tr = car.tr;
    lf = car.lf;      lr = car.lr;
    h_cog = car.h_cog;   
    h_rc_f = car.h_rc_f;    h_rc_r = car.h_rc_r;

    % IR_FR = kin(1);   IR_FL = kin(2);
    % IR_RR = kin(3);    IR_RL = kin(4);
    % 
    % tf = kin(5);      tr = kin(6);
    % lf = kin(7);      lr = kin(8);
    % h_cog = kin(9);   
    % h_rc_f = kin(10);    h_rc_r = kin(11);

    % MEZZE CARREGGIATE
    t_f = tf / 2;
    t_r = tr / 2;

    % --- UNPACKING AERODINAMICA ---
    Cz   = aero_coeffs(1);
    Cx   = aero_coeffs(2);
    x_cp = aero_coeffs(3);

    L = lf + lr;
    g = 9.81;
    ms  = car.m_sprung; Iyy = car.Iyy; Ixx = car.Ixx;
    muf = car.m_unsprung_F; mur = car.m_unsprung_R;

    % --- 3. RIGIDEZZE EQUIVALENTI ALLA RUOTA ---
    IR_f_avg = (IR_FR + IR_FL) / 2;
    IR_r_avg = (IR_RR + IR_RL) / 2;
    IR = [IR_f_avg; IR_f_avg; IR_r_avg; IR_r_avg];

    ksf = car.k_spring_front * 1000 * IR_f_avg^2; 
    ksr = car.k_spring_rear  * 1000 * IR_r_avg^2;  
    ktf = car.k_tyre_front   * 1000; 
    ktr = car.k_tyre_rear    * 1000;

    % Le barre prendono i valori normali. L'approccio esplicito le rende sicure.
    kabf = car.k_ARB_front; 
    kabr = car.k_ARB_rear;  

    % --- 4. CINEMATICA TELAIO (Altezze e Velocità degli attacchi) ---
    z_chassis_FL = q(1) - lf*q(2) + t_f*q(3);
    z_chassis_FR = q(1) - lf*q(2) - t_f*q(3);
    z_chassis_RL = q(1) + lr*q(2) + t_r*q(3);
    z_chassis_RR = q(1) + lr*q(2) - t_r*q(3);

    v_chassis_FL = dq(1) - lf*dq(2) + t_f*dq(3);
    v_chassis_FR = dq(1) - lf*dq(2) - t_f*dq(3);
    v_chassis_RL = dq(1) + lr*dq(2) + t_r*dq(3);
    v_chassis_RR = dq(1) + lr*dq(2) - t_r*dq(3);

    % Corner Ride Heights (Daltezze libere da terra)
    corner_rh = [car.h0_ground_front + z_chassis_FR; 
                 car.h0_ground_front + z_chassis_FL; 
                 car.h0_ground_rear  + z_chassis_RR; 
                 car.h0_ground_rear  + z_chassis_RL];

    % Velocità di compressione ammortizzatore
    susp_vel_ground = [dq(5) - v_chassis_FR; 
                       dq(4) - v_chassis_FL; 
                       dq(7) - v_chassis_RR; 
                       dq(6) - v_chassis_RL];

    % --- 5. COMPRESSIONE SOSPENSIONI ---
    % delta_z: compressione della sospensione (Positivo = ruota più vicina al telaio)
    delta_z_FL = q(4) - z_chassis_FL;
    delta_z_FR = q(5) - z_chassis_FR;
    delta_z_RL = q(6) - z_chassis_RL;
    delta_z_RR = q(7) - z_chassis_RR;

    % --- 6. FORZE SOSPENSIONI ---
    % 1. Forze Molle
    F_spring_FL = ksf * delta_z_FL;
    F_spring_FR = ksf * delta_z_FR;
    F_spring_RL = ksr * delta_z_RL;
    F_spring_RR = ksr * delta_z_RR;

    % 2. Forze Barre Antirollio (Differenza di compressione sullo stesso asse)
    F_arb_FL = kabf * (delta_z_FL - delta_z_FR);
    F_arb_FR = kabf * (delta_z_FR - delta_z_FL);
    F_arb_RL = kabr * (delta_z_RL - delta_z_RR);
    F_arb_RR = kabr * (delta_z_RR - delta_z_RL);

    % 3. Forze Damper (Input dalla tua lookup table)
    F_d_FR = F_damp_in(1);
    F_d_FL = F_damp_in(2);
    F_d_RR = F_damp_in(3);
    F_d_RL = F_damp_in(4);

    % FORZA TOTALE DELLA SOSPENSIONE SUL TELAIO
    F_susp_FL = F_spring_FL + F_arb_FL + F_d_FL;
    F_susp_FR = F_spring_FR + F_arb_FR + F_d_FR;
    F_susp_RL = F_spring_RL + F_arb_RL + F_d_RL;
    F_susp_RR = F_spring_RR + F_arb_RR + F_d_RR;

    % --- 7. FORZANTI ESTERNE ---
    Downforce = 0.5 * car.rho * car.frontal_area * Cz * (u^2);
    Drag      = 0.5 * car.rho * car.frontal_area * Cx * (u^2);

    M_aero_pitch = -Drag * (car.h_cp - h_cog) + Downforce * (lf - x_cp);
    M_pitch_ext  = -(car.m * ax_prev * h_cog) + M_aero_pitch;

    h_rc = (h_rc_f * lr + h_rc_r * lf) / L;
    M_roll_ext   = (car.m * ay_prev * (h_cog - h_rc));

    % --- 8. RISOLUZIONE MODELLO (EQUAZIONI DIFFERENZIALI) ---
    % A. MASSA SOSPESA (Telaio)
    sum_Fz_chassis = F_susp_FL + F_susp_FR + F_susp_RL + F_susp_RR - Downforce;
    sum_M_pitch    = -(F_susp_FL + F_susp_FR)*lf + (F_susp_RL + F_susp_RR)*lr + M_pitch_ext;
    sum_M_roll     =  (F_susp_FL - F_susp_FR)*t_f + (F_susp_RL - F_susp_RR)*t_r + M_roll_ext;

    ddq_heave = sum_Fz_chassis / ms;
    ddq_pitch = sum_M_pitch / Iyy;
    ddq_roll  = sum_M_roll / Ixx;

    % B. MASSE NON SOSPESE (Ruote)
    % La gomma spinge la ruota verso l'alto
    F_tyre_FL = -ktf * q(4);
    F_tyre_FR = -ktf * q(5);
    F_tyre_RL = -ktr * q(6);
    F_tyre_RR = -ktr * q(7);

    % La sospensione spinge la ruota in verso opposto rispetto a come spinge il telaio
    ddq_uFL = (F_tyre_FL - F_susp_FL) / muf;
    ddq_uFR = (F_tyre_FR - F_susp_FR) / muf;
    ddq_uRL = (F_tyre_RL - F_susp_RL) / mur;
    ddq_uRR = (F_tyre_RR - F_susp_RR) / mur;

    % Ricompattamento
    ddq = [ddq_heave; ddq_pitch; ddq_roll; ddq_uFL; ddq_uFR; ddq_uRL; ddq_uRR];
    dx  = [dq; ddq];

    % --- 9. CALCOLO FZ A TERRA ---
    delta_Fz_geom_front = (car.m * ay_prev * (lr / L) * h_rc_f) / tf;
    delta_Fz_geom_rear  = (car.m * ay_prev * (lf / L) * h_rc_r) / tr;

    delta_Fz_inertia  = (2 * Jr_tot + 2 * car.J_f) * ax_prev / (car.R * L);
    delta_Fz_roll_res = (car.m * g + Downforce) * car.rolling_resistance / L;

    Fz_stat_f = (car.m * g * lr / L) / 2;
    Fz_stat_r = (car.m * g * lf / L) / 2;

    Fz_FR = Fz_stat_f - ktf * q(5) + delta_Fz_geom_front - delta_Fz_inertia - delta_Fz_roll_res; 
    Fz_FL = Fz_stat_f - ktf * q(4) - delta_Fz_geom_front - delta_Fz_inertia - delta_Fz_roll_res; 
    Fz_RR = Fz_stat_r - ktr * q(7) + delta_Fz_geom_rear  + delta_Fz_inertia + delta_Fz_roll_res; 
    Fz_RL = Fz_stat_r - ktr * q(6) - delta_Fz_geom_rear  + delta_Fz_inertia + delta_Fz_roll_res; 

    Fz = [Fz_FR; Fz_FL; Fz_RR; Fz_RL];
    Fz(Fz < 0) = 0; 

    % --- 10. OUTPUT CINEMATICI FINALI (Con Virtual Rails) ---

    wheel_travel = [delta_z_FR; 
                    delta_z_FL; 
                    delta_z_RR; 
                    delta_z_RL] * 1000; 
    
    tyre_deflection = [Fz(1) / ktf;
                       Fz(2) / ktf;
                       Fz(3) / ktr;
                       Fz(4) / ktr];
end

== matlab function Vehicle_definitivo_validazione_2/Driver in the Loop/Vehicle/Powertrain/Electric Motor/MATLAB Function ==
  data: T_FR input; T_FL input; w_FR input; w_FL input; SoC input; SoC_dot output
function SoC_dot  = fcn_Battery(T_FR, T_FL, w_FR, w_FL, SoC)
    
    % --- 1. PARAMETRI BATTERIA E POWERTRAIN ---
    C_Ah = 50; % Capacità totale del pacco batteria in Ah (es. accumulatore FS)
    n_cells_series = 100; % Numero di celle collegate in serie
    eta_em = 0.95; % Efficienza combinata Motore + Inverter
    P_aux = 500;   % [Watt] Potenza costantemente assorbita dai servizi (pompe, LV, ECU)
    
    % --- 2. CURVE CARATTERISTICHE (Dipendenti dal SoC) ---
    % Approssimazione lineare per cella Li-ion: da 3.0V (scarica) a 4.2V (carica)
    OCV_cell = 3.0 + (1.2 * SoC); 
    Rin_cell = 0.005; % Resistenza interna della singola cella [Ohm]
    
    V_oc = OCV_cell * n_cells_series; % Tensione a vuoto dell'intero pacco
    R_in = Rin_cell * n_cells_series; % Resistenza interna totale
    
    % --- 3. POTENZA ELETTRICA MOTORE 1 ---
    P_mech1 = T_FR * w_FR;
    if P_mech1 >= 0
        P_elec1 = P_mech1 / eta_em; % Trazione: assorbe più di quanto eroga
    else
        P_elec1 = P_mech1 * eta_em; % Rigenerazione: immette meno di quanto frena
    end
    
    % --- 4. POTENZA ELETTRICA MOTORE 2 ---
    P_mech2 = T_FL * w_FL;
    if P_mech2 >= 0
        P_elec2 = P_mech2 / eta_em; % Trazione
    else
        P_elec2 = P_mech2 * eta_em; % Rigenerazione
    end
    
    % --- 5. CARICO ELETTRICO TOTALE SULLA BATTERIA ---
    % La batteria vede la somma algebrica dei due inverter più i servizi
    P_tot_elec = P_elec1 + P_elec2 + P_aux;
    
    % --- 6. CALCOLO CORRENTE E TENSIONE (CIRCUITO EQUIVALENTE) ---
    % Risoluzione dell'equazione di 2° grado: Rin * I^2 - Voc * I + P_tot = 0
    discriminante = V_oc^2 - 4 * R_in * P_tot_elec;
    
    if discriminante < 0
        % Protezione numerica: la richiesta di potenza supera il limite fisico
        % della batteria (il voltage sag la manderebbe a zero). 
        % Eroga la corrente massima teorica (Cortocircuito).
        I_batt = V_oc / (2 * R_in); 
    else
        % Soluzione standard per la corrente prelevata (o immessa se P_tot < 0)
        I_batt = (V_oc - sqrt(discriminante)) / (2 * R_in);
    end
    
    % Voltaggio reale ai morsetti (al netto del Voltage Sag)
    V_batt = V_oc - R_in * I_batt;
    
    % Potenza dissipata per effetto Joule (utile per dimensionare il raffreddamento)
    P_dissipata = R_in * (I_batt^2);
    
    % --- 7. DERIVATA DELLO STATE OF CHARGE (Coulomb Counting) ---
    % SoC_dot [1/s]. I_batt è in Ampere (C/s), la capacità si porta in Coulomb (*3600)
    SoC_dot = -I_batt / (C_Ah * 3600);
    
end

== matlab function Vehicle_definitivo_validazione_2/Driver in the Loop/Vehicle/Powertrain/pwt con clutch/Differential1 ==
  data: T_rear input; T_RR output; w_RR input; w_RL input; T_RL output; car input
function [T_RR, T_RL] = fcn_Salisbury_LSD(T_rear, w_RR, w_RL, car)
   
    % Coefficienti di smoothing (Stabilità Simulink)
    k_blend = 10; 
    k_slip  = 5; 
    
    % --- 2. TRANSIZIONE POWER-ON / POWER-OFF (Senza IF) ---
    w_blend = 0.5 * (1 + tanh(k_blend * T_rear));
    mu_active = car.mu_Poff + (car.mu_Pon - car.mu_Poff) * w_blend;
    
    % --- 3. CALCOLO CAPACITÀ DI BLOCCAGGIO (Mf_max) ---
    T_ramps = mu_active * abs(T_rear);
    Mf_max = max(car.Mf_preload, T_ramps); 
    
    % --- 4. APPLICAZIONE COPPIA ATTRITO (Modello Continuo) ---
    delta_w = w_RR - w_RL; 
    T_lock = Mf_max * tanh(k_slip * delta_w);
    
    % --- 5. RIPARTIZIONE FINALE ---
    % Se w_RR è maggiore (delta_w > 0, T_lock > 0), tolgo a RR e do a RL
    T_RR = (T_rear / 2) - T_lock;
    T_RL = (T_rear / 2) + T_lock;
end

== matlab function Vehicle_definitivo_validazione_2/Driver in the Loop/Vehicle/Powertrain/pwt con clutch/MATLAB Function1 ==
  data: w_ice input; condizione output; w_rear input
function condizione = fcn(w_ice, w_rear)
    
if (w_ice - w_rear) < 50
    condizione = true;
else
    condizione = false;
end

end

== matlab function Vehicle_definitivo_validazione_2/Driver in the Loop/Vehicle/Powertrain/pwt con clutch/MATLAB Function4 ==
  data: u input; next_gear output; tps input; bps input; current_gear input; shift_timer_in input; shift_timer_out output; torque_mult output
function [next_gear, shift_timer_out, torque_mult] = Gearbox_ECU(u, tps, bps, current_gear, shift_timer_in)
   
    dt = 0.001;               
    shift_duration = 0.030;   
    nGearMax = 4;             
    
    v_thresh_up   = [0, 24.9444, 29.1, inf]; 
    v_thresh_down = [0, 18, 26.5, 29.5];
    
    % Inizializzazione sicura
    % if current_gear == 0
    %     current_gear = 2; % Partenza in 2° marcia
    % end
    
    next_gear = current_gear;
    
    if shift_timer_in > 0
        torque_mult = 0;                           
        shift_timer_out = shift_timer_in - dt;     
    else
        torque_mult = 1;                           
        shift_timer_out = 0;                       
        if current_gear < nGearMax && u >= v_thresh_up(current_gear) && tps > 0 && bps == 0
            next_gear = current_gear + 1;
            shift_timer_out = shift_duration;                  
        elseif current_gear > 1 && u <= v_thresh_down(current_gear) && (bps > 0 || tps == 0)
            next_gear = current_gear - 1;
            shift_timer_out = shift_duration;      
        end
    end
end

== matlab function Vehicle_definitivo_validazione_2/Senza relaxation/Vehicle/Powertrain/pwt senza clutch/Gearbox ==
  data: u input; next_gear output; torque_mult output; tps input; bps input; current_gear input; shift_timer_in input; shift_timer_out output
function [next_gear, torque_mult, shift_timer_out] = Gearbox_ECU(u, tps, bps, current_gear, shift_timer_in)
   
    dt = 0.001;               
    shift_duration = 0.030;   
    nGearMax = 4;             
    
    v_thresh_up   = [0, 24.9444, 29.1, inf]; 
    v_thresh_down = [0, 18, 26.5, 29.5];
    
    % Inizializzazione sicura
    % if current_gear == 0
    %     current_gear = 2; % Partenza in 2° marcia
    % end
    
    next_gear = current_gear;
    
    if shift_timer_in > 0
        torque_mult = 0;                           
        shift_timer_out = shift_timer_in - dt;     
    else
        torque_mult = 1;                           
        shift_timer_out = 0;                       
        if current_gear < nGearMax && u >= v_thresh_up(current_gear) && tps > 0 && bps == 0
            next_gear = current_gear + 1;
            shift_timer_out = shift_duration;                  
        elseif current_gear > 1 && u <= v_thresh_down(current_gear) && (bps > 0 || tps == 0)
            next_gear = current_gear - 1;
            shift_timer_out = shift_duration;      
        end
    end
end
